simulink model "Part3_2"  (R2021b)
settings: Solver=VariableStepAuto  StartTime=0.0  StopTime=10.0  RelTol=1e-3
settings Model: Creator=Matin  LastModifiedBy=Matin

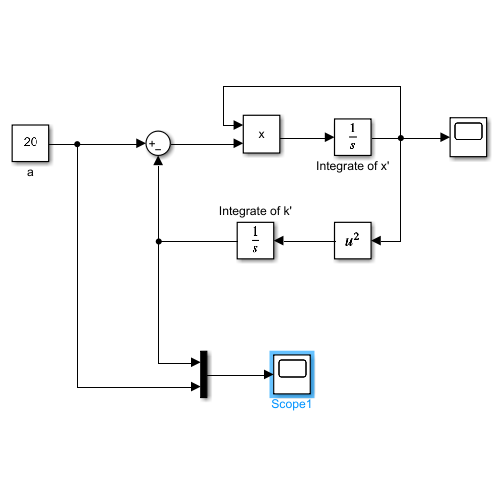
[thumbnail: Simulink's stored preview of the top-level diagram]
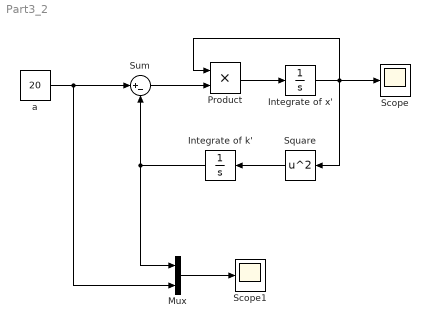
== system Part3_2 ==
  Integrate of k' : Integrator
  Integrate of x' : Integrator  InitialCondition=20
  Mux : Mux  Inputs=2
  Product : Product
  Scope : Scope
  Scope1 : Scope
  Square : Math  Operator=square  SaturateOnIntegerOverflow=on
  Sum : Sum  Inputs=|+-
  a : Constant  Value=20
  wires:
  a/1 -> Mux/2, Sum/1
  Sum/1 -> Product/2
  Product/1 -> Integrate of x'/1
  Integrate of x'/1 -> Square/1, Product/1, Scope/1
  Square/1 -> Integrate of k'/1
  Integrate of k'/1 -> Sum/2, Mux/1
  Mux/1 -> Scope1/1
